simulink model "HESS_SC_Active_new"  (R2014a)
settings: Solver=ode45  StartTime=0.0  StopTime=1370  RelTol=1e-3
values from neighbouring files (symbols this model uses):
  Cap_cell = 2000    [Run_Simulink.m]
  Current_dot2C = 0.2*Current_1C    (= 17.6)    [Run_Simulink.m]
  Current_dot5C = 0.5*Current_1C    (= 44)    [Run_Simulink.m]
  Current_limitation = Current_dot8C    (= 70.4)    [Run_Simulink.m]
  SC_numbers = 113    [Run_Simulink.m]
  V_C_100 = 305    [Run_Simulink.m]
  V_C_25 = 152.5    [Run_Simulink.m]
  V_C_50 = 215.6    [Run_Simulink.m]
  V_C_75 = 264    [Run_Simulink.m]
  Vol_cell = 2.7    [Run_Simulink.m]
undefined symbols (not defined in the file or in its folder): Ion, Lithium
libraries: powerlib x12, electricdrivelib x1
settings Model: Creator=Administrator  LastModifiedBy=Administrator
settings SolverCC: AlgebraicLoopSolver=LineSearch

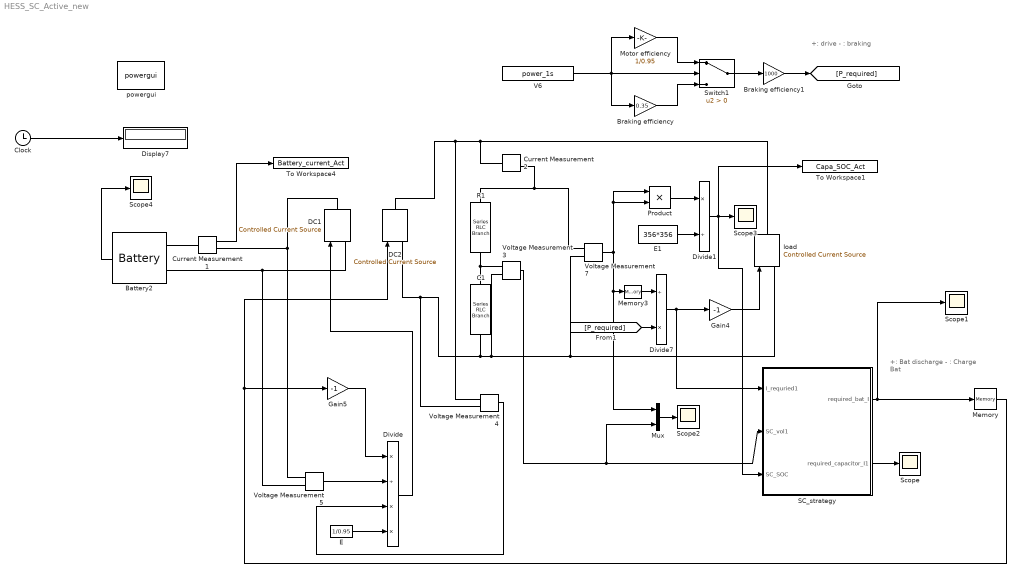
== system HESS_SC_Active_new ==
  note: +: Bat discharge
      | - : Charge Bat
  note: +: drive
      | - : braking
  Battery2 : electricdrivelib/Extra Sources/Battery  BatType=Lithium-Ion  ShowDetailedParameters=on  NomV=259.25  NomQ=88  SOC=90  PresetModel=on  MaxQ=88  FullV=301.7637  Dis_rate=38.2609  R=0.02946  Normal_OP=79.5826  expZone="[280.09      4.323478]"  Dis_Char=off  current=[1.5 3]  Units=Ampere-hour  Batt_Tr=30
  Braking efficiency : Gain  Gain=0.35
  Braking efficiency1 : Gain  Gain=1000
  C1 : powerlib/Elements/Series RLC Branch  LConnTagsString=__new0  RConnTagsString=__new0  BranchType=C  Resistance=1  Inductance=1e-3  SetiL0=off  InitialCurrent=0  Capacitance=Cap_cell/SC_numbers  Setx0=on  InitialVoltage=Vol_cell*SC_numbers  Measurements=Branch voltage
  Clock : Clock
  Current Measurement1 : powerlib/Measurements/Current Measurement  PhasorSimulation=off  OutputType=Complex  PSBequivalent=0
  Current Measurement2 : powerlib/Measurements/Current Measurement  PhasorSimulation=off  OutputType=Complex  PSBequivalent=0
  DC1 : powerlib/Electrical Sources/Controlled Current Source  Initialize=on  Source_Type=AC  Amplitude=0  Phase=0  Frequency=0  Measurements=None
  DC2 : powerlib/Electrical Sources/Controlled Current Source  Initialize=on  Source_Type=AC  Amplitude=0  Phase=0  Frequency=0  Measurements=None
  Display7 : Display
  Divide : Product  Inputs=*/**
  Divide1 : Product  Inputs=*/
  Divide7 : Product  Inputs=/*
  E : Constant  Value=1/0.95
  E1 : Constant  Value=356*356
  Gain4 : Gain  Gain=-1
  Gain5 : Gain  Gain=-1
  Memory : Memory
  Memory3 : Memory  X0=380
  Motor efficiency : Gain  Gain=1/0.95
  Mux : Mux  Inputs=2
  Product : Product
  R1 : powerlib/Elements/Series RLC Branch  LConnTagsString=__new0  RConnTagsString=__new0  BranchType=R  Resistance=0.0462  Inductance=1e-3  SetiL0=off  InitialCurrent=0  Capacitance=1e-6  Setx0=off  InitialVoltage=0  Measurements=None
  SC_strategy : Subsystem
  Scope{,1..4} (5 alike) : Scope
      Scope2 settings: TimeRange=1600  YMin=240  YMax=420  SaveName=ScopeData2
      Scope3 settings: SaveName=ScopeData4
      Scope4 settings: SaveName=ScopeData3
  Switch1 : Switch  Criteria=u2 > Threshold
  To Workspace1 : ToWorkspace  VariableName=Capa_SOC_Act  SampleTime=-1
  To Workspace4 : ToWorkspace  VariableName=Battery_current_Act  SampleTime=-1
  V6 : FromWorkspace  VariableName=power_1s  SampleTime=1
  Voltage Measurement{3..5,7} (4 alike) : powerlib/Measurements/Voltage Measurement  PhasorSimulation=off  OutputType=Complex  PSBequivalent=0
  load : powerlib/Electrical Sources/Controlled Current Source  Initialize=on  Source_Type=AC  Amplitude=0  Phase=0  Frequency=0  Measurements=None
  powergui : powerlib/powergui  Priority=1  SimulationMode=Discrete  SolverType=Tustin  SampleTime=1  frequency=60  SPID=off  DisableSnubberDevices=off  DisableRonSwitches=off  DisableVfSwitches=off  SwTol=0  Interpol=off  DisplayEquations=off  Ts=0  methode=off  frequencyindice=0  Pbase=100e6  ErrMax=1e-4  Iterations=50  UnitsV=kV  UnitsW=MW  FunctionMessages=off  echomessages=off  HookPort=off  EnableUseOfTLC=off  x0status=blocks  RestoreLinks=warning  ResistiveCurrentMeasurement=off  Frange=[0:2:500]  Ylog=off  Xlog=on  ShowGrid=off  save=off  variable=ZData  structure=0  ZoomFFT=off  StartTime=0.0  cycles=1  DisplayStyle=1  fundamental=60  FreqAxis=off  MaxFrequency=1000  frequencyindicesteady=1  RmsSteady=1  display=off
  wires:
  Clock/1 -> Display7/1
  Divide7/1 -> Gain4/1, SC_strategy/1(I_requried1)
  Battery2/1 -> Scope4/1
  Voltage Measurement4/1 -> Divide/3
  Voltage Measurement3/1 -> SC_strategy/2(SC_vol1), Mux/2
  E/1 -> Divide/4
  Voltage Measurement5/1 -> Divide/2
  Divide/1 -> DC1/1
  SC_strategy/1(required_bat_I) -> Scope1/1, Memory/1
  Memory/1 -> DC2/1, Gain5/1
  Gain5/1 -> Divide/1
  [P_required] -> Divide7/2
  Voltage Measurement7/1 -> Mux/1, Memory3/1, Product/2, Product/1
  Memory3/1 -> Divide7/1
  Mux/1 -> Scope2/1
  V6/1 -> Motor efficiency/1, Braking efficiency/1, Switch1/2
  Motor efficiency/1 -> Switch1/1
  Braking efficiency/1 -> Switch1/3
  Switch1/1 -> Braking efficiency1/1
  Current Measurement1/1 -> To Workspace4/1
  Gain4/1 -> load/1
  SC_strategy/2(required_capacitor_I1) -> Scope/1
  Braking efficiency1/1 -> [P_required]
  Product/1 -> Divide1/1
  E1/1 -> Divide1/2
  Divide1/1 -> SC_strategy/3(SC_SOC), To Workspace1/1, Scope3/1
  connections:
  load/RConn1 -- Current Measurement2/LConn1 -- Voltage Measurement4/LConn1 -- DC2/RConn1
  Voltage Measurement3/LConn1 -- R1/RConn1 -- C1/LConn1
  Voltage Measurement7/LConn2 -- load/LConn1 -- Voltage Measurement3/LConn2 -- DC2/LConn1 -- Voltage Measurement4/LConn2 -- C1/RConn1
  Voltage Measurement5/LConn1 -- Current Measurement1/RConn1 -- DC1/RConn1
  Voltage Measurement5/LConn2 -- DC1/LConn1 -- Battery2/LConn2
  Current Measurement2/RConn1 -- R1/LConn1 -- Voltage Measurement7/LConn1
  Battery2/LConn1 -- Current Measurement1/LConn1

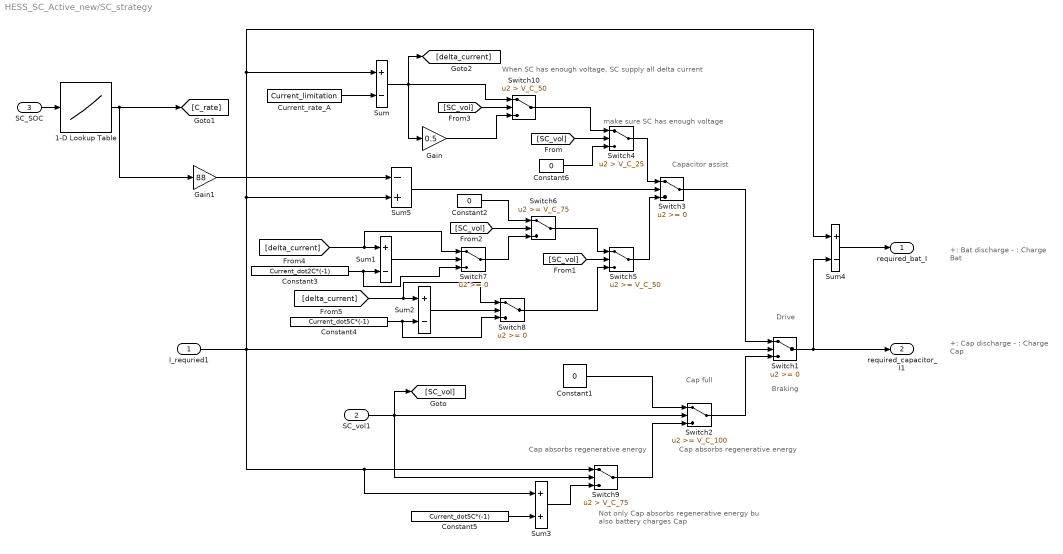
== system HESS_SC_Active_new/SC_strategy ==
  note: +: Cap discharge
      | - : Charge Cap
  note: Capacitor assist
  note: Braking
  note: Drive
  note: Cap full
  note: Cap absorbs regenerative energy
  note: make sure SC has enough voltage
  note: Not only Cap absorbs regenerative energy
      | bu also battery charges Cap
  note: Cap absorbs regenerative energy
  note: +: Bat discharge
      | - : Charge Bat
  note: When SC has enough voltage, SC supply all delta current
  I_requried1 : Inport
  SC_vol1 : Inport  Port=2
  SC_SOC : Inport  Port=3
  1-D Lookup Table : Lookup_n-D  NumberOfTableDimensions=1  BreakpointsForDimension1=[0.25,0.6,1]  Table=[0.8,0.5,0.15]  InternalRulePriority=Speed  RndMeth=Simplest  InputSameDT=on
  Constant1 : Constant  Value=0
  Constant2 : Constant  Value=0
  Constant3 : Constant  Value=Current_dot2C*(-1)
  Constant4 : Constant  Value=Current_dot5C*(-1)
  Constant5 : Constant  Value=Current_dot5C*(-1)
  Constant6 : Constant  Value=0
  Current_rate_A : Constant  Value=Current_limitation
  Gain : Gain  Gain=0.5
  Gain1 : Gain  Gain=88
  Sum{,1..2,4} (4 alike) : Sum  Inputs=+-
  Sum3 : Sum
  Sum5 : Sum  Inputs=-+
  Switch{1,3,7..8} (4 alike) : Switch
  Switch10 : Switch  Criteria=u2 > Threshold  Threshold=V_C_50
  Switch2 : Switch  Threshold=V_C_100
  Switch4 : Switch  Criteria=u2 > Threshold  Threshold=V_C_25
  Switch5 : Switch  Threshold=V_C_50
  Switch6 : Switch  Threshold=V_C_75
  Switch9 : Switch  Criteria=u2 > Threshold  Threshold=V_C_75
  required_bat_I : Outport
  required_capacitor_I1 : Outport  Port=2
  wires:
  I_requried1/1 -> Switch1/2, Switch9/1, Sum3/1, Sum4/1, Sum/1, Sum5/2
  Constant1/1 -> Switch2/1
  Switch1/1 -> Sum4/2, required_capacitor_I1/1
  Switch2/1 -> Switch1/3
  Current_rate_A/1 -> Sum/2
  Switch3/1 -> Switch1/1
  SC_vol1/1 -> Switch9/2, [SC_vol], Switch2/2
  [SC_vol] -> Switch4/2
  Sum/1 -> Gain/1, Switch10/1, [delta_current]
  Switch4/1 -> Switch3/1
  Switch5/1 -> Switch3/3
  [SC_vol] -> Switch5/2
  [SC_vol] -> Switch6/2
  Constant2/1 -> Switch6/1
  Switch6/1 -> Switch5/1
  Switch8/1 -> Switch5/3
  [delta_current] -> Switch7/1, Sum1/1
  Constant3/1 -> Switch7/3, Sum1/2
  Sum1/1 -> Switch7/2
  Switch7/1 -> Switch6/3
  [delta_current] -> Sum2/1, Switch8/1
  Constant4/1 -> Sum2/2, Switch8/3
  Sum2/1 -> Switch8/2
  Constant5/1 -> Sum3/2
  Sum3/1 -> Switch9/3
  Switch9/1 -> Switch2/3
  Constant6/1 -> Switch4/3
  Sum4/1 -> required_bat_I/1
  [SC_vol] -> Switch10/2
  Gain/1 -> Switch10/3
  Switch10/1 -> Switch4/1
  SC_SOC/1 -> 1-D Lookup Table/1
  1-D Lookup Table/1 -> [C_rate], Gain1/1
  Gain1/1 -> Sum5/1
  Sum5/1 -> Switch3/2
